simulink model "mod3"  (Simulink 7.9)
settings: Solver=ode45  StartTime=0.0  StopTime=simu.trantime  RelTol=1e-3
undefined symbols (not defined in the file): dc, Fs, mod, OSR, sinamp, sinfreq
libraries: dspsigops x4, dsparch4 x1, simulink x1, dspsrcs4 x1
settings Model: Creator=Isacco Arnaldi  LastModifiedBy=Arnaldi Isacco
settings SolverCC: AutoInsertRateTranBlk=on
settings DataIOCC: MaxDataPoints=50000  SaveOutput=off  SaveTime=off
settings DebuggingCC: StrictBusMsg=Warning
settings CodeAppCC: CustomSymbolStrType=$N$R$M_T
settings GRTTargetCC: CombineOutputUpdateFcns=off  GRTInterface=on

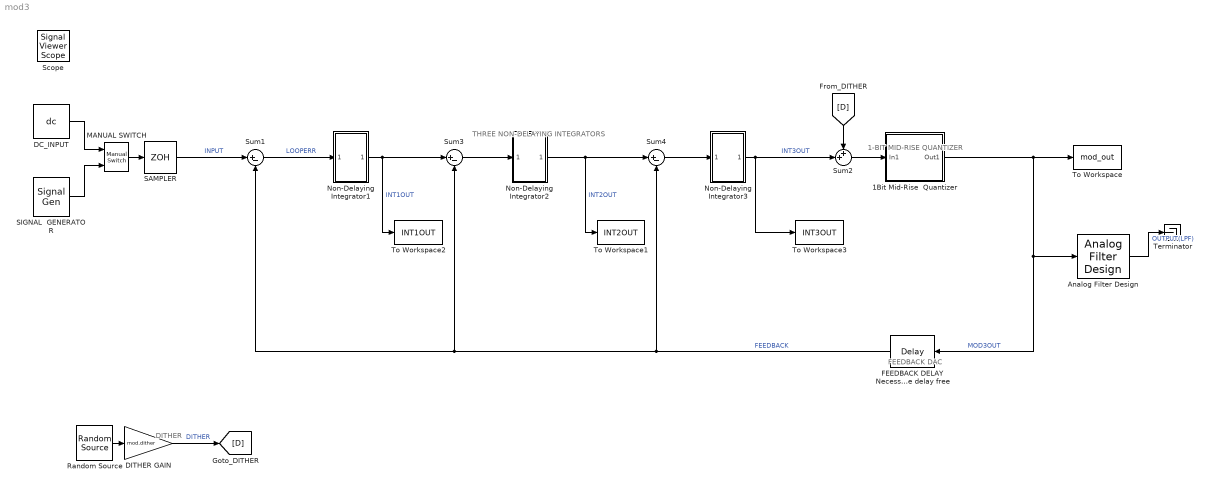
== system mod3 ==
  note: THREE NON-DELAYING
      |  INTEGRATORS
  note: FEEDBACK DAC
  note: 1-BIT  MID-RISE
      | QUANTIZER
  note: DITHER
  1Bit Mid-Rise  Quantizer : Subsystem
  Analog Filter Design : dsparch4/Analog Filter Design  method=Butterworth  filttype=Lowpass  N=8  Wlo=pi*(Fs/OSR)  Whi=80  Rp=2  Rs=40
      settings: AttributesFormatString=Low-pass filter the loop output\nto illustrate intuitively how the\npulse density modulated +1/-1\noutput stream does indeed capture\nthe input signal
  DC_INPUT : Constant  Value=dc  VectorParams1D=off  OutDataTypeStr=double  SampleTime=1/Fs
  DITHER GAIN : Gain  Gain=mod.dither  SampleTime=1/Fs
  FEEDBACK DELAY Necessary to avoid a delay-free loop as integrator and quantizer are delay free : dspsigops/Delay  InputProcessing=Inherited (this choice will be removed - see release notes)  dly_unit=Samples  delay=1  ic_detail=off  dif_ic_for_ch=off  dif_ic_for_dly=off  ic=0  reset_popup=None
  MANUAL SWITCH : simulink/Signal Routing/Manual Switch  sw=1  action=0  varsize=off
      settings: AttributesFormatString=Double click to\nselect the desired\ninput
  Non-Delaying Integrator1 : Subsystem
  Non-Delaying Integrator2 : Subsystem
  Non-Delaying Integrator3 : Subsystem
  Random Source : dspsrcs4/Random Source  SrcType=Uniform  NormMethod=Ziggurat  CltLength=12  MinVal=-1  MaxVal=1  MeanVal=0  VarVal=1  RepMode=Not repeatable  rawSeed=1  IsInherit=off  SampMode=Discrete  SampTime=1/Fs  SampFrame=1  DataType=Double  OutComplex=Real
  SAMPLER : ZeroOrderHold  SampleTime=1/Fs
  SIGNAL  GENERATOR : SignalGenerator  Amplitude=sinamp  Frequency=sinfreq  VectorParams1D=off
  Sum1 : Sum  Inputs=|+-  SampleTime=1/Fs
      settings: AttributesFormatString=Modulator Input\nLoop Error (input - fbk)
  Sum2 : Sum  Inputs=++|
  Sum3 : Sum  Inputs=|+-
  Sum4 : Sum  Inputs=|+-
  Terminator : Terminator
  To Workspace : ToWorkspace  VariableName=mod_out  SampleTime=-1
      settings: AttributesFormatString=Export output to\nworkspace for\npost-processing
  To Workspace1 : ToWorkspace  VariableName=INT2OUT  SampleTime=-1
  To Workspace2 : ToWorkspace  VariableName=INT1OUT  SampleTime=-1
  To Workspace3 : ToWorkspace  VariableName=INT3OUT  SampleTime=-1
  Scope : SignalViewerScope  IOType=viewer  NumInputPorts=5  RefreshTime=0.035000
      settings: YMin=-5~-5~-5~-5~-5  YMax=5~5~5~5~5
  wires:
  Sum1/1 -> Non-Delaying Integrator1/1(In1)  "LOOPERR"
  Random Source/1 -> DITHER GAIN/1
  DITHER GAIN/1 -> [D]  "DITHER"
  DC_INPUT/1 -> MANUAL SWITCH/1
  SIGNAL  GENERATOR/1 -> MANUAL SWITCH/2
  MANUAL SWITCH/1 -> SAMPLER/1
  Analog Filter Design/1 -> Terminator/1  "OUTPUT(LPF)"
  Sum2/1 -> 1Bit Mid-Rise  Quantizer/1(In1)
  [D] -> Sum2/1
  1Bit Mid-Rise  Quantizer/1(Out1) -> To Workspace/1, Analog Filter Design/1, FEEDBACK DELAY Necessary to avoid a delay-free loop as integrator and quantizer are delay free/1  "MOD3OUT"
  SAMPLER/1 -> Sum1/1  "INPUT"
  Non-Delaying Integrator1/1(Out1) -> Sum3/1, To Workspace2/1  "INT1OUT"
  Non-Delaying Integrator2/1(Out1) -> Sum4/1, To Workspace1/1  "INT2OUT"
  Sum3/1 -> Non-Delaying Integrator2/1(In1)
  Sum4/1 -> Non-Delaying Integrator3/1(In1)
  Non-Delaying Integrator3/1(Out1) -> Sum2/2, To Workspace3/1  "INT3OUT"
  FEEDBACK DELAY Necessary to avoid a delay-free loop as integrator and quantizer are delay free/1 -> Sum1/2, Sum3/2, Sum4/2  "FEEDBACK"

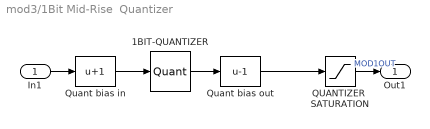
== system mod3/1Bit Mid-Rise  Quantizer ==
  In1 : Inport
  1BIT-QUANTIZER : Quantizer  QuantizationInterval=2  LinearizeAsGain=off  SampleTime=1/Fs
      settings: AttributesFormatString=step = 2
  QUANTIZER  SATURATION : Saturate  UpperLimit=mod.qsatout1  LowerLimit=-(mod.qsatout1)
      settings: AttributesFormatString=Limit quantizer\noutput
  Quant bias in : Bias  Bias=1
      settings: AttributesFormatString=Need offset to give\nMID-RISE quantiser
  Quant bias out : Bias  Bias=-1
      settings: AttributesFormatString=Shift outputs to\n..., -2, 1, 1, ...
  Out1 : Outport
  wires:
  Quant bias out/1 -> QUANTIZER  SATURATION/1
  Quant bias in/1 -> 1BIT-QUANTIZER/1
  1BIT-QUANTIZER/1 -> Quant bias out/1
  QUANTIZER  SATURATION/1 -> Out1/1  "MOD1OUT"
  In1/1 -> Quant bias in/1

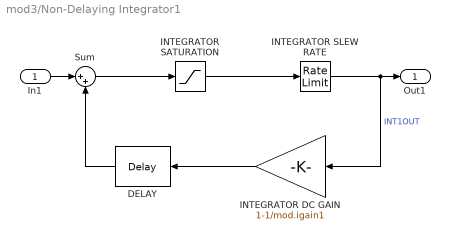
== system mod3/Non-Delaying Integrator1 ==
  In1 : Inport
  DELAY : dspsigops/Delay  InputProcessing=Inherited (this choice will be removed - see release notes)  dly_unit=Samples  delay=1  ic_detail=off  dif_ic_for_ch=off  dif_ic_for_dly=off  ic=0  reset_popup=None
  INTEGRATOR SATURATION : Saturate  UpperLimit=mod.isat1  LowerLimit=-(mod.isat1)
      settings: AttributesFormatString=Real integrators will have\noutput swing limits (analog\nsignal headroom or digital\naccumulator min/max values)
  INTEGRATOR SLEW RATE : RateLimiter  RisingSlewLimit=mod.isr1  FallingSlewLimit=-(mod.isr1)  SampleTimeMode=inherited
      settings: AttributesFormatString=...and\nmay suffer from\npoor slew rate
  INTEGRATOR DC GAIN : Gain  Gain=1-1/mod.igain1
      settings: AttributesFormatString=Integrator leakage\n(model finite integrator dc/LF\ngain in analog modulators)
  Sum : Sum  Inputs=|++
      settings: AttributesFormatString=Integrator\nsummer
  Out1 : Outport
  wires:
  DELAY/1 -> Sum/2
  Sum/1 -> INTEGRATOR SATURATION/1
  INTEGRATOR DC GAIN/1 -> DELAY/1
  INTEGRATOR SLEW RATE/1 -> INTEGRATOR DC GAIN/1, Out1/1  "INT1OUT"
  INTEGRATOR SATURATION/1 -> INTEGRATOR SLEW RATE/1
  In1/1 -> Sum/1

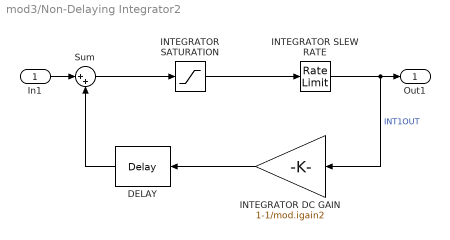
== system mod3/Non-Delaying Integrator2 ==
  In1 : Inport
  DELAY : dspsigops/Delay  InputProcessing=Inherited (this choice will be removed - see release notes)  dly_unit=Samples  delay=1  ic_detail=off  dif_ic_for_ch=off  dif_ic_for_dly=off  ic=0  reset_popup=None
  INTEGRATOR SATURATION : Saturate  UpperLimit=mod.isat2  LowerLimit=-(mod.isat2)
      settings: AttributesFormatString=Real integrators will have\noutput swing limits (analog\nsignal headroom or digital\naccumulator min/max values)
  INTEGRATOR SLEW RATE : RateLimiter  RisingSlewLimit=mod.isr2  FallingSlewLimit=-(mod.isr2)  SampleTimeMode=inherited
      settings: AttributesFormatString=...and\nmay suffer from\npoor slew rate
  INTEGRATOR DC GAIN : Gain  Gain=1-1/mod.igain2
      settings: AttributesFormatString=Integrator leakage\n(model finite integrator dc/LF\ngain in analog modulators)
  Sum : Sum  Inputs=|++
      settings: AttributesFormatString=Integrator\nsummer
  Out1 : Outport
  wires:
  DELAY/1 -> Sum/2
  Sum/1 -> INTEGRATOR SATURATION/1
  INTEGRATOR DC GAIN/1 -> DELAY/1
  INTEGRATOR SLEW RATE/1 -> INTEGRATOR DC GAIN/1, Out1/1  "INT1OUT"
  INTEGRATOR SATURATION/1 -> INTEGRATOR SLEW RATE/1
  In1/1 -> Sum/1

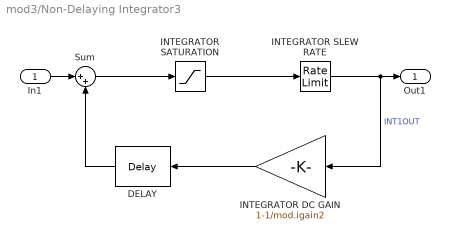
== system mod3/Non-Delaying Integrator3 ==
  In1 : Inport
  DELAY : dspsigops/Delay  InputProcessing=Inherited (this choice will be removed - see release notes)  dly_unit=Samples  delay=1  ic_detail=off  dif_ic_for_ch=off  dif_ic_for_dly=off  ic=0  reset_popup=None
  INTEGRATOR SATURATION : Saturate  UpperLimit=mod.isat2  LowerLimit=-(mod.isat2)
      settings: AttributesFormatString=Real integrators will have\noutput swing limits (analog\nsignal headroom or digital\naccumulator min/max values)
  INTEGRATOR SLEW RATE : RateLimiter  RisingSlewLimit=mod.isr2  FallingSlewLimit=-(mod.isr2)  SampleTimeMode=inherited
      settings: AttributesFormatString=...and\nmay suffer from\npoor slew rate
  INTEGRATOR DC GAIN : Gain  Gain=1-1/mod.igain2
      settings: AttributesFormatString=Integrator leakage\n(model finite integrator dc/LF\ngain in analog modulators)
  Sum : Sum  Inputs=|++
      settings: AttributesFormatString=Integrator\nsummer
  Out1 : Outport
  wires:
  DELAY/1 -> Sum/2
  Sum/1 -> INTEGRATOR SATURATION/1
  INTEGRATOR DC GAIN/1 -> DELAY/1
  INTEGRATOR SLEW RATE/1 -> INTEGRATOR DC GAIN/1, Out1/1  "INT1OUT"
  INTEGRATOR SATURATION/1 -> INTEGRATOR SLEW RATE/1
  In1/1 -> Sum/1
